simulink model "CAR_MODEL"  (R2023a)
settings: Solver=VariableStepAuto  StartTime=0.0  StopTime=10.0  RelTol=1e-3
undefined symbols (not defined in the file or in its folder): MODEL_INI
settings Model: Creator=juanluiszamora  LastModifiedBy=juanluiszamora
settings SolverCC: AlgebraicLoopSolver=TrustRegion
settings DataIOCC: ReturnWorkspaceOutputs=off
settings DebuggingCC: UnconnectedInputMsg=warning  UnconnectedOutputMsg=warning  UnconnectedLineMsg=warning  PregeneratedLibrarySubsystemCodeDiagnostic=none  InitInArrayFormatMsg=none  ArithmeticOperatorsInVariantConditions=warning
settings ModelReferenceCC: EnableRefExpFcnMdlSchedulingChecks=on
settings SFSimCC: SimUseLocalCustomCode=off  CustomCodeUndefinedFunction=UseInterfaceOnly
settings RTWCC: RTWUseLocalCustomCode=off  DLArmComputeVersion=19.05

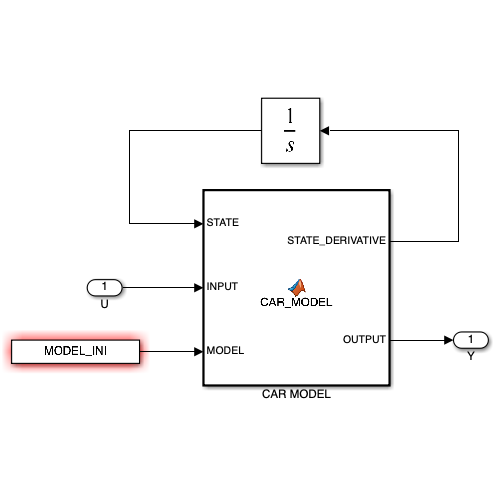
[thumbnail: Simulink's stored preview of the top-level diagram]
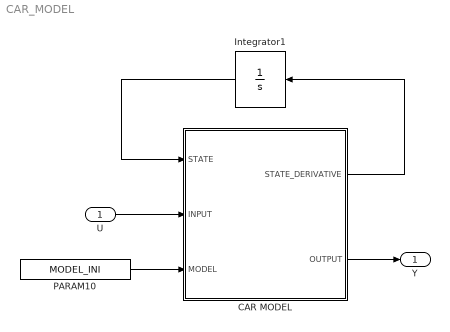
== system CAR_MODEL ==
  U : Inport  PortDimensions=2
  CAR MODEL : MATLAB Function  TreatAsAtomicUnit=on
  Integrator1 : Integrator  InitialCondition=zeros(6,1)
  PARAM10 : Constant  Value=MODEL_INI  OutDataTypeStr=Bus: MODEL_Bus  SampleTime=0
  Y : Outport  VectorParamsAs1DForOutWhenUnconnected=off
  wires:
  CAR MODEL/2(OUTPUT) -> Y/1
  Integrator1/1 -> CAR MODEL/1(STATE)
  PARAM10/1 -> CAR MODEL/3(MODEL)
  CAR MODEL/1(STATE_DERIVATIVE) -> Integrator1/1
  U/1 -> CAR MODEL/2(INPUT)

== matlab function CAR_MODEL/CAR MODEL ==
  data: STATE input; INPUT input; STATE_DERIVATIVE output; OUTPUT output; MODEL input
function [STATE_DERIVATIVE,OUTPUT] = CAR_MODEL(STATE,INPUT,MODEL)

%% Reference frames
% Fixed or earth reference frame
% X,e1I - North
% Y,e2I - East
% Z,e3I - Down
% Body reference frame with origin in the center of mass
% Xb,e1B - forward axis
% Yb,e2B - right axis
% Zb,e3B - downward axis

%--------------------------------------------------------------
% MOTOR PARAMETERS
%--------------------------------------------------------------
% Rotor resistance (ohm)
Rm = MODEL.PARAM.MOTOR_RESISTANCE;
% Motor back-emf constant (V/rad*s)
Ke = MODEL.PARAM.MOTOR_BEMF_CONSTANT;
% Torque constant (N.m/A)
Kt = MODEL.PARAM.MOTOR_TORQUE_CONSTANT;
% Motor static torque (N. m) eje motor
Trmax = 0*MODEL.PARAM.MOTOR_STATIC_TORQUE; 
% Viscous friction coefficient in the motor axis (N.m.s/rad)
Dm = MODEL.PARAM.MOTOR_VISCOUS_FRICTION_COEFF;
% Motor + wheel inertia in the motor axis (kg.m^2)
Im = MODEL.PARAM.MOTOR_INERTIA;
% Motor gear ratio
n1 = MODEL.PARAM.MOTOR_GEAR_RATIO;

%--------------------------------------------------------------
% CAR PARAMETERS
%--------------------------------------------------------------
% Body mass without wheels (kg)
M = MODEL.PARAM.BODY_MASS; 
% Wheel mass including the rotor (kg)
m = MODEL.PARAM.WHEEL_MASS;
% Body inertia in x-axis (kg.m^2)
Ix = MODEL.PARAM.BODY_INERTIA_X;
% Body inertia in y-axis (pitch) (kg.m^2)
Iy = MODEL.PARAM.BODY_INERTIA_Y;
% Body inertia in z-axis (kg.m^2)
Iz = MODEL.PARAM.BODY_INERTIA_Z;
% Viscous friction coefficient in x-axis (N.m.s/rad)
Dx = MODEL.PARAM.BODY_VISCOUS_FRICTION_COEFF_X;
% Viscous friction coefficient in z-axis (N.m.s/rad)
Dz = MODEL.PARAM.BODY_VISCOUS_FRICTION_COEFF_Z;
% Center of gravity distance from the wheel axis (m)
h = MODEL.PARAM.BODY_DISTANCE;
% Wheel radius (m)
R = MODEL.PARAM.WHEEL_RADIUS;
% Distance between wheels (m)
W = MODEL.PARAM.WHEEL_DISTANCE;
% Wheel gear ratio 
n2 = MODEL.PARAM.WHEEL_GEAR_RATIO; 

%--------------------------------------------------------------
% OTHER PARAMETERS
%--------------------------------------------------------------
% Gravity (m/s^2)
g = MODEL.PARAM.GRAVITY;
% Vehicle mode: / 0. CAR / 1. SELF-BALANCING VEHICLE
vmode = MODEL.PARAM.VEHICLE_MODE;
% Yaw and range sensor parameters
if vmode == 0 % CAR
    Iyaw = Iz;
    Dyaw = Dz;
    if MODEL.PARAM.WALL_FOLLOWER_MODE
        xA = MODEL.PARAM.LIDAR_2D_XA;
        yA = MODEL.PARAM.LIDAR_2D_YA;        
    else
        xA = MODEL.PARAM.RANGE_XA;
        yA = MODEL.PARAM.RANGE_YA;
    end
else % SELF-BALANCING VEHICLE
    Iyaw = Ix;
    Dyaw = Dx;
    xA = MODEL.PARAM.RANGE_ZA;
    yA = MODEL.PARAM.RANGE_YA;  
end

%--------------------------------------------------------------
% STATE VARIABLES
%--------------------------------------------------------------
% Forward velocity (m/s)
vc = STATE(1);
% Yaw rate (rad/s)
dShi = STATE(2);
% Yaw angle (rad)
Shi = STATE(3);
% Wall distance (m)
% d_wall = STATE(4);
% Pitch rate (rad/s)
dTheta = STATE(5);
% Pitch angle (rad)
Theta = STATE(6);

%--------------------------------------------------------------
% INPUT VARIABLES
%--------------------------------------------------------------
% Motor voltages (V)
ul = INPUT(1);
ur = INPUT(2);

%%%%%%%%%%%%%%%%%%%%%%%%%%%%%%%%%%%%%%%%%%%%%%%%%%%%%%%%%%%%%%%%%%%%%%%%%%%
% STATE EQUATIONS
%%%%%%%%%%%%%%%%%%%%%%%%%%%%%%%%%%%%%%%%%%%%%%%%%%%%%%%%%%%%%%%%%%%%%%%%%%%
%--------------------------------------------------------------
% Differential velocity of the wheels (m/s)
vd = W/2*dShi;
% Common angular rate of the wheels (rad/s)
wc = vc/R;
% Differential angular rate of the wheels (rad/s)
wd = vd/R;
%--------------------------------------------------------------
% Common angular rate of the motors (rad/s)
wmc = n2*wc + dTheta/n1;
% Differential angular rate of the motors (rad/s)
wmd = n2*wd;
%--------------------------------------------------------------
% Motor rate 
wml = wmc + wmd;
wmr = wmc - wmd;
% wmc = (wmr+wml)/2;
% wmd = (wml-wmr)/2
%--------------------------------------------------------------
% Motor equations
el = Ke*wml;
er = Ke*wmr;
% dil = (ul - el - Rm*il)/Lm;
% dir = (ur - er - Rm*ir)/Lm;
% Currents
il = (ul - el)/Rm;
ir = (ur - er)/Rm;
% Motor torques
Tml = Kt*il;
Tmr = Kt*ir;
Tmc = (Tml+Tmr)/2;
Tmd = (Tml-Tmr)/2;
%--------------------------------------------------------------
% Static friction torques
Trl_lim = Tml*(abs(Tml)<Trmax) - Trmax*(Tml<=-Trmax) + Trmax*(Tml>=Trmax);
Trl = Trl_lim*(abs(wml)==0) + Trmax*sign(wml)*(abs(wml)>0);
Trr_lim = Tmr*(abs(Tmr)<Trmax) - Trmax*(Tmr<=-Trmax) + Trmax*(Tmr>=Trmax);
Trr = Trr_lim*(abs(wmr)==0) + Trmax*sign(wmr)*(abs(wmr)>0);
Trc = (Trl+Trr)/2;
Trd = (Trl-Trr)/2;
%--------------------------------------------------------------
% Viscous friction torques
Tdl = Dm*wml;
Tdr = Dm*wmr;
Tdc = (Tdr+Tdl)/2;
Tdd = (Tdl-Tdr)/2;
%--------------------------------------------------------------
% Total motor torque
% Tl = Tml - Tdl - Trl - Frl*R/n2;
% Tr = Tmr - Tdr - Trr - Frr*R/n2;
% Tc = (Tl+Tr)/2;
%--------------------------------------------------------------
% Motor angular accelerations
% dwml = Tl/Im = (Tml-Tdl-Trl-Frl*R/n2)/Im
% dwmr = Tr/Im = (Tmr-Tdr-Trr-Frr*R/n2)/Im
%--------------------------------------------------------------
% Friction body forces
% Frl = n2/R*(Tml-Tdl-Trl-Im*dwml)
% Frr = n2/R*(Tmr-Tdr-Trr-Im*dwmr)
%--------------------------------------------------------------
if vmode == 0
    %--------------------------------------------------------------
    % Translation equation in x-axis
    % Frl + Frr = (M+2*m)*dvc
    % 2*n2/R*(Tmc-Tdc-Trc) = (M+2*m+2*(n2/R)^2*Im)*dvc
    %---------------------------------------------------------    %--------------------------------------------------------------
    % Computation of dvc (CAR)
    dvc = 2*n2/R*(Tmc-Tdc-Trc)/(M+2*m+2*(n2/R)^2*Im);
    d2Theta = 0;
    % (M+2*m+2*(n2/R)^2*Im)*dvc + 2*n2^2/R^2*(Dm+Kt*Ke/Rm)*vc = 2*n2*Kt/R/Rm*uc
    % Tv*dvc + vc = Kv*uc
    % Kv = 2*n2*Kt/R/Rm/(2*(n2/R)^2*(Dm+Kt*Ke/Rm))
    % Tv = (M+2*m+2*(n2/R)^2*Im)/(2*(n2/R)^2*(Dm+Kt*Ke/Rm))
    %--------------------------------------------------------------
else
    %--------------------------------------------------------------
    % Translation equation in x-axis
    % Frl + Frr = (M+2*m)*dvc  - M*h*cos(Theta)*d2Theta + M*h*sin(Theta)*dTheta^2
    % 2*n2/R*(Tmc-Tdc-Trc) - M*h*sin(Theta)*dTheta^2 =
    %    = (M+2*m+2*(n2/R)^2*Im)*dvc  - (M*h*cos(Theta)-2*n2/n1/R*Im)*d2Theta
    %--------------------------------------------------------------
    % Chassis reaction force Nx
    % Nx - M*g*sin(Theta) = M*cos(Theta)*dvc - M*h*d2Theta
    % h*Nx + 2/n1*Tc = Iy*d2Theta
    % Nx = M*cos(Theta)*dvc - M*h*d2Theta + M*g*sin(Theta)
    % M*g*h*sin(Theta) + M*h*cos(Theta)*dvc - M*h^2*d2Theta + 2*Tc = Iy*d2Theta
    % 2/n1*Tc + M*g*h*sin(Theta) = -M*h*cos(Theta)*dvc + (Iy+M*h^2)*d2Theta
    % M*g*h*sin(Theta) = -(M*h*cos(Theta)+2*n2/n1/R*Im)*dvc + (Iy+M*h^2-2*Im/n1^2)*d2Theta
    %--------------------------------------------------------------
    % Computation of dvc and d2Theta (SELF-BALANCING VEHICLE)
    matA = [       M+2*m+2*(n2/R)^2*Im      -(M*h*cos(Theta)-2*n2/n1/R*Im)
        -(M*h*cos(Theta)+2*n2/n1/R*Im)        Iy+M*h^2-2*Im/n1^2      ];
    matB = [   2*n2/R*(Tmc-Tdc-Trc)+M*h*dTheta^2*sin(Theta)
        M*g*h*sin(Theta) ];
    aux = matA\matB;
    dvc = aux(1);
    d2Theta = aux(2);
    %--------------------------------------------------------------
end
%--------------------------------------------------------------% Rotation equation in z-axis
% Rotation equation in yaw-axis
% Frl - Frr = 2*n2/R*(Tmd-Tdd-Trd-Im*dwmd)
% Torque in yaw-axis (earth reference-frame)
% Tz = (Frl-Frr)*W/2 - Dyaw*dShi
% Iyaw*d2Shi = W/2*(Frl-Frr) - Dyaw*dShi
% Iyaw*d2Shi = n2*W/R*(Tmd-Tdd-Trd-Im*dwmd) - Dyaw*dShi
% wmd = n2*wd = n2/R*vd = n2*W/2/R*dShi
% dwmd = W/R/2*d2Shi
% Iyaw*d2Shi = n2*W/R*(Tmd-Tdd-Trd-Im*n2*W/R/2*d2Shi) - Dyaw*dShi
% (Iyaw+(n2*W/R)^2/2*Im)*d2Shi = n2*W/R*(Tmd-Tdd-Trd) - Dyaw*dShi
d2Shi = 1/(Iyaw+(n2*W/R)^2/2*Im)*(n2*W/R*(Tmd-Tdd-Trd) - Dyaw*dShi);
% (Iyaw+(n2*W/R)^2/2*Im)*d2Shi + Dyaw*dShi + n2*W/R*Tdd  = n2*W/R/Rm*Kt*(ud-ed)
% (Iz+n2*(W/R)^2/2*Im)*d2Shi + Dz*dShi + n2^2/R^2*W^2/2*Dm*dShi + n2^2/R^2*W^2/2*Kt*Ke/Rm*dShi = n2*W/R/Rm*Kt*ud
% Kw = n2/R*W*Kt/Rm/(Dyaw+n2^2/R^2*W^2/2*(Dm+Kt*Ke/Rm))
% Tw = (Iyaw+(n2*W/R)^2/2*Im)/(Dyaw+n2^2/R^2*W^2/2*(Dm+Kt*Ke/R
%--------------------------------------------------------------
% Wall follower
dd_wall = -(vc-dShi*yA)*sin(Shi) - dShi*xA*cos(Shi);

%%%%%%%%%%%%%%%%%%%%%%%%%%%%%%%%%%%%%%%%%%%%%%%%%%%%%%%%%%%%%%%%%%%%%%%%%%%
STATE_DERIVATIVE = [dvc ; d2Shi ; dShi ; dd_wall ; d2Theta ; dTheta];
%%%%%%%%%%%%%%%%%%%%%%%%%%%%%%%%%%%%%%%%%%%%%%%%%%%%%%%%%%%%%%%%%%%%%%%%%%%

%%%%%%%%%%%%%%%%%%%%%%%%%%%%%%%%%%%%%%%%%%%%%%%%%%%%%%%%%%%%%%%%%%%%%%%%%%%
% OUTPUT BUS
%%%%%%%%%%%%%%%%%%%%%%%%%%%%%%%%%%%%%%%%%%%%%%%%%%%%%%%%%%%%%%%%%%%%%%%%%%%
OUTPUT = STATE;

return
